simulink model "EPA_Walker"  (R2018a)
settings: Solver=FixedStepDiscrete  StartTime=0.0  StopTime=inf  FixedStep=0.001  RelTol=1e-3  EnableMultiTasking=on
model workspace (MAT data in the model file):
  MCOS : class17 (value not decoded)
undefined symbols (not defined in the file or in its folder): bits_current, bits_GRF, bits_Kd, bits_Kp, bits_position, bits_velocity, deadzone_in_TIB, deadzone_out_TIB, GRF_MAX, GRF_MIN, k_p_TIB, KD_MAX, KD_MIN, KP_MAX, KP_MIN, P_MAX, P_MIN, PressureFilter_CutOffFreq, PressureFilter_Gain, ReadingVoltage, T_MAX, T_MIN, V_MAX, V_MIN, voltageBias_GAS, voltageBias_GL, voltageBias_HAM, voltageBias_IL, voltageBias_POP, voltageBias_RF, voltageBias_SOL, voltageBias_TIB, voltageBias_VAS, voltageMultiplier_GAS, voltageMultiplier_GL, voltageMultiplier_HAM, voltageMultiplier_IL, voltageMultiplier_POP, voltageMultiplier_RF, voltageMultiplier_SOL, voltageMultiplier_TIB, voltageMultiplier_VAS, VoltageResolution
libraries: xpcethercatlib x139, simulink x19, peGeneralControl x18, slrtlib x9
(part 3 of 5)

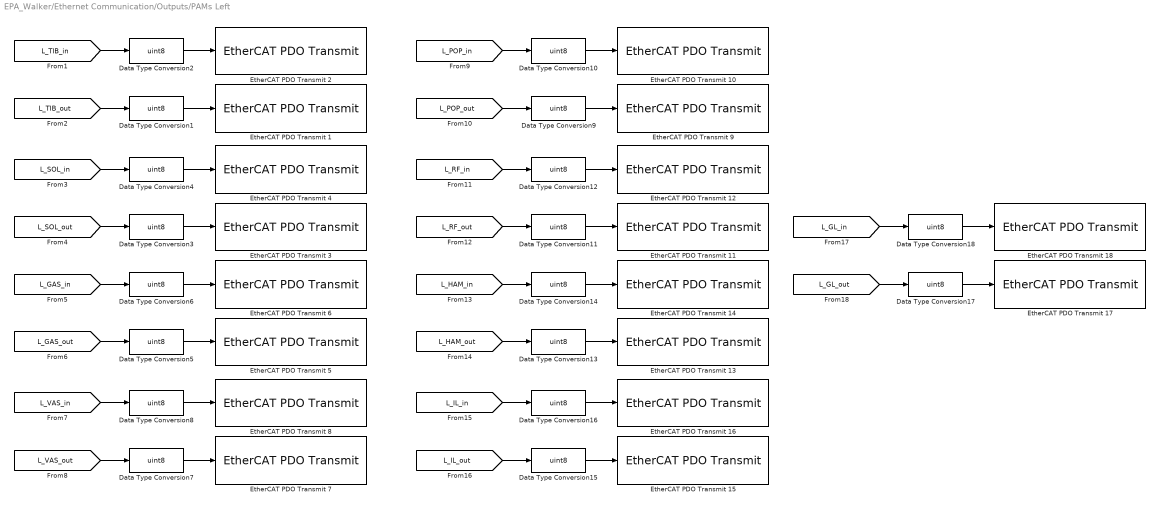
== system EPA_Walker/Ethernet Communication/Outputs/PAMs Left ==
  Data Type Conversion{1..18} (18 alike) : DataTypeConversion  OutDataTypeStr=uint8  RndMeth=Ceiling
  EtherCAT PDO Transmit 1 : xpcethercatlib/EtherCAT PDO Transmit   Priority=3  sig_name=PAMs_L.Outputs.Byte1  sig_offset=1032  sig_type=uint8  type_size=8  sig_dim=1  device_id=0  sample_time=0.001000
      settings: SourceProductName=Simulink Real-Time  SourceProductBaseCode=XP
  EtherCAT PDO Transmit 10 : xpcethercatlib/EtherCAT PDO Transmit   Priority=3  sig_name=PAMs_L.Outputs.Byte8  sig_offset=1088  sig_type=uint8  type_size=8  sig_dim=1  device_id=0  sample_time=0.001000
      settings: SourceProductName=Simulink Real-Time  SourceProductBaseCode=XP
  EtherCAT PDO Transmit 11 : xpcethercatlib/EtherCAT PDO Transmit   Priority=3  sig_name=PAMs_L.Outputs.Byte11  sig_offset=1112  sig_type=uint8  type_size=8  sig_dim=1  device_id=0  sample_time=0.001000
      settings: SourceProductName=Simulink Real-Time  SourceProductBaseCode=XP
  EtherCAT PDO Transmit 12 : xpcethercatlib/EtherCAT PDO Transmit   Priority=3  sig_name=PAMs_L.Outputs.Byte10  sig_offset=1104  sig_type=uint8  type_size=8  sig_dim=1  device_id=0  sample_time=0.001000
      settings: SourceProductName=Simulink Real-Time  SourceProductBaseCode=XP
  EtherCAT PDO Transmit 13 : xpcethercatlib/EtherCAT PDO Transmit   Priority=3  sig_name=PAMs_L.Outputs.Byte13  sig_offset=1128  sig_type=uint8  type_size=8  sig_dim=1  device_id=0  sample_time=0.001000
      settings: SourceProductName=Simulink Real-Time  SourceProductBaseCode=XP
  EtherCAT PDO Transmit 14 : xpcethercatlib/EtherCAT PDO Transmit   Priority=3  sig_name=PAMs_L.Outputs.Byte12  sig_offset=1120  sig_type=uint8  type_size=8  sig_dim=1  device_id=0  sample_time=0.001000
      settings: SourceProductName=Simulink Real-Time  SourceProductBaseCode=XP
  EtherCAT PDO Transmit 15 : xpcethercatlib/EtherCAT PDO Transmit   Priority=3  sig_name=PAMs_L.Outputs.Byte15  sig_offset=1144  sig_type=uint8  type_size=8  sig_dim=1  device_id=0  sample_time=0.001000
      settings: SourceProductName=Simulink Real-Time  SourceProductBaseCode=XP
  EtherCAT PDO Transmit 16 : xpcethercatlib/EtherCAT PDO Transmit   Priority=3  sig_name=PAMs_L.Outputs.Byte14  sig_offset=1136  sig_type=uint8  type_size=8  sig_dim=1  device_id=0  sample_time=0.001000
      settings: SourceProductName=Simulink Real-Time  SourceProductBaseCode=XP
  EtherCAT PDO Transmit 17 : xpcethercatlib/EtherCAT PDO Transmit   Priority=3  sig_name=PAMs_L.Outputs.Byte17  sig_offset=1160  sig_type=uint8  type_size=8  sig_dim=1  device_id=0  sample_time=0.001000
      settings: SourceProductName=Simulink Real-Time  SourceProductBaseCode=XP
  EtherCAT PDO Transmit 18 : xpcethercatlib/EtherCAT PDO Transmit   Priority=3  sig_name=PAMs_L.Outputs.Byte16  sig_offset=1152  sig_type=uint8  type_size=8  sig_dim=1  device_id=0  sample_time=0.001000
      settings: SourceProductName=Simulink Real-Time  SourceProductBaseCode=XP
  EtherCAT PDO Transmit 2 : xpcethercatlib/EtherCAT PDO Transmit   Priority=3  sig_name=PAMs_L.Outputs.Byte0  sig_offset=1024  sig_type=uint8  type_size=8  sig_dim=1  device_id=0  sample_time=0.001000
      settings: SourceProductName=Simulink Real-Time  SourceProductBaseCode=XP
  EtherCAT PDO Transmit 3 : xpcethercatlib/EtherCAT PDO Transmit   Priority=3  sig_name=PAMs_L.Outputs.Byte3  sig_offset=1048  sig_type=uint8  type_size=8  sig_dim=1  device_id=0  sample_time=0.001000
      settings: SourceProductName=Simulink Real-Time  SourceProductBaseCode=XP
  EtherCAT PDO Transmit 4 : xpcethercatlib/EtherCAT PDO Transmit   Priority=3  sig_name=PAMs_L.Outputs.Byte2  sig_offset=1040  sig_type=uint8  type_size=8  sig_dim=1  device_id=0  sample_time=0.001000
      settings: SourceProductName=Simulink Real-Time  SourceProductBaseCode=XP
  EtherCAT PDO Transmit 5 : xpcethercatlib/EtherCAT PDO Transmit   Priority=3  sig_name=PAMs_L.Outputs.Byte5  sig_offset=1064  sig_type=uint8  type_size=8  sig_dim=1  device_id=0  sample_time=0.001000
      settings: SourceProductName=Simulink Real-Time  SourceProductBaseCode=XP
  EtherCAT PDO Transmit 6 : xpcethercatlib/EtherCAT PDO Transmit   Priority=3  sig_name=PAMs_L.Outputs.Byte4  sig_offset=1056  sig_type=uint8  type_size=8  sig_dim=1  device_id=0  sample_time=0.001000
      settings: SourceProductName=Simulink Real-Time  SourceProductBaseCode=XP
  EtherCAT PDO Transmit 7 : xpcethercatlib/EtherCAT PDO Transmit   Priority=3  sig_name=PAMs_L.Outputs.Byte7  sig_offset=1080  sig_type=uint8  type_size=8  sig_dim=1  device_id=0  sample_time=0.001000
      settings: SourceProductName=Simulink Real-Time  SourceProductBaseCode=XP
  EtherCAT PDO Transmit 8 : xpcethercatlib/EtherCAT PDO Transmit   Priority=3  sig_name=PAMs_L.Outputs.Byte6  sig_offset=1072  sig_type=uint8  type_size=8  sig_dim=1  device_id=0  sample_time=0.001000
      settings: SourceProductName=Simulink Real-Time  SourceProductBaseCode=XP
  EtherCAT PDO Transmit 9 : xpcethercatlib/EtherCAT PDO Transmit   Priority=3  sig_name=PAMs_L.Outputs.Byte9  sig_offset=1096  sig_type=uint8  type_size=8  sig_dim=1  device_id=0  sample_time=0.001000
      settings: SourceProductName=Simulink Real-Time  SourceProductBaseCode=XP
  wires:
  Data Type Conversion2/1 -> EtherCAT PDO Transmit 2/1
  [L_TIB_in] -> Data Type Conversion2/1
  [L_TIB_out] -> Data Type Conversion1/1
  Data Type Conversion1/1 -> EtherCAT PDO Transmit 1/1
  Data Type Conversion3/1 -> EtherCAT PDO Transmit 3/1
  [L_SOL_in] -> Data Type Conversion4/1
  [L_SOL_out] -> Data Type Conversion3/1
  Data Type Conversion4/1 -> EtherCAT PDO Transmit 4/1
  Data Type Conversion6/1 -> EtherCAT PDO Transmit 6/1
  Data Type Conversion8/1 -> EtherCAT PDO Transmit 8/1
  [L_VAS_out] -> Data Type Conversion7/1
  [L_GAS_in] -> Data Type Conversion6/1
  [L_GAS_out] -> Data Type Conversion5/1
  [L_VAS_in] -> Data Type Conversion8/1
  Data Type Conversion7/1 -> EtherCAT PDO Transmit 7/1
  Data Type Conversion5/1 -> EtherCAT PDO Transmit 5/1
  [L_IL_in] -> Data Type Conversion16/1
  Data Type Conversion16/1 -> EtherCAT PDO Transmit 16/1
  Data Type Conversion13/1 -> EtherCAT PDO Transmit 13/1
  [L_HAM_out] -> Data Type Conversion13/1
  [L_IL_out] -> Data Type Conversion15/1
  [L_HAM_in] -> Data Type Conversion14/1
  Data Type Conversion14/1 -> EtherCAT PDO Transmit 14/1
  Data Type Conversion10/1 -> EtherCAT PDO Transmit 10/1
  Data Type Conversion12/1 -> EtherCAT PDO Transmit 12/1
  [L_RF_out] -> Data Type Conversion11/1
  [L_POP_in] -> Data Type Conversion10/1
  Data Type Conversion15/1 -> EtherCAT PDO Transmit 15/1
  [L_POP_out] -> Data Type Conversion9/1
  [L_RF_in] -> Data Type Conversion12/1
  Data Type Conversion11/1 -> EtherCAT PDO Transmit 11/1
  Data Type Conversion9/1 -> EtherCAT PDO Transmit 9/1
  Data Type Conversion17/1 -> EtherCAT PDO Transmit 17/1
  [L_GL_in] -> Data Type Conversion18/1
  [L_GL_out] -> Data Type Conversion17/1
  Data Type Conversion18/1 -> EtherCAT PDO Transmit 18/1

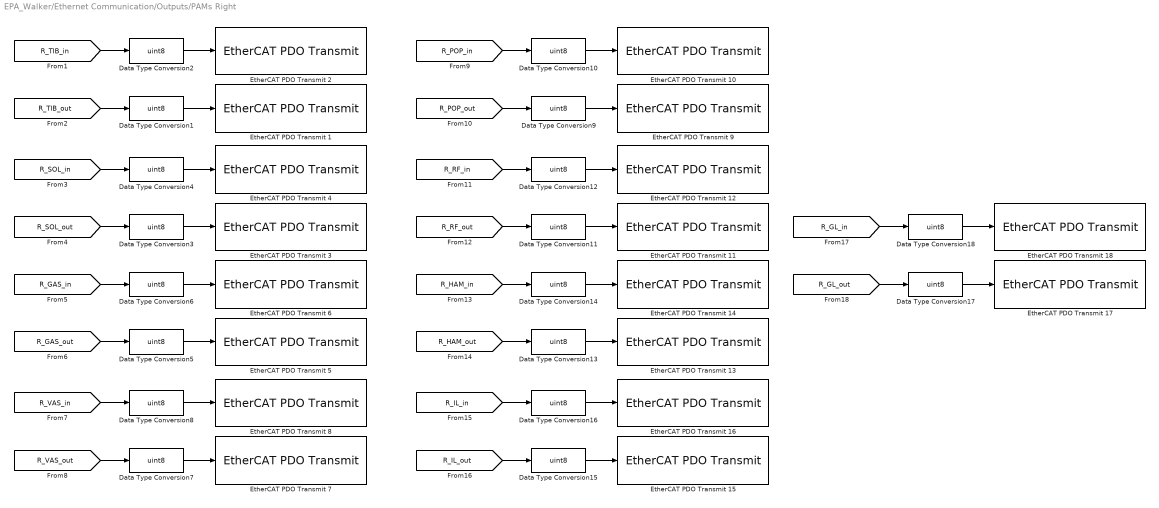
== system EPA_Walker/Ethernet Communication/Outputs/PAMs Right ==
  Data Type Conversion{1..18} (18 alike) : DataTypeConversion  OutDataTypeStr=uint8  RndMeth=Ceiling
  EtherCAT PDO Transmit 1 : xpcethercatlib/EtherCAT PDO Transmit   Priority=3  sig_name=PAMs_R.Outputs.Byte1  sig_offset=520  sig_type=uint8  type_size=8  sig_dim=1  device_id=0  sample_time=0.001000
      settings: SourceProductName=Simulink Real-Time  SourceProductBaseCode=XP
  EtherCAT PDO Transmit 10 : xpcethercatlib/EtherCAT PDO Transmit   Priority=3  sig_name=PAMs_R.Outputs.Byte8  sig_offset=576  sig_type=uint8  type_size=8  sig_dim=1  device_id=0  sample_time=0.001000
      settings: SourceProductName=Simulink Real-Time  SourceProductBaseCode=XP
  EtherCAT PDO Transmit 11 : xpcethercatlib/EtherCAT PDO Transmit   Priority=3  sig_name=PAMs_R.Outputs.Byte11  sig_offset=600  sig_type=uint8  type_size=8  sig_dim=1  device_id=0  sample_time=0.001000
      settings: SourceProductName=Simulink Real-Time  SourceProductBaseCode=XP
  EtherCAT PDO Transmit 12 : xpcethercatlib/EtherCAT PDO Transmit   Priority=3  sig_name=PAMs_R.Outputs.Byte10  sig_offset=592  sig_type=uint8  type_size=8  sig_dim=1  device_id=0  sample_time=0.001000
      settings: SourceProductName=Simulink Real-Time  SourceProductBaseCode=XP
  EtherCAT PDO Transmit 13 : xpcethercatlib/EtherCAT PDO Transmit   Priority=3  sig_name=PAMs_R.Outputs.Byte13  sig_offset=616  sig_type=uint8  type_size=8  sig_dim=1  device_id=0  sample_time=0.001000
      settings: SourceProductName=Simulink Real-Time  SourceProductBaseCode=XP
  EtherCAT PDO Transmit 14 : xpcethercatlib/EtherCAT PDO Transmit   Priority=3  sig_name=PAMs_R.Outputs.Byte12  sig_offset=608  sig_type=uint8  type_size=8  sig_dim=1  device_id=0  sample_time=0.001000
      settings: SourceProductName=Simulink Real-Time  SourceProductBaseCode=XP
  EtherCAT PDO Transmit 15 : xpcethercatlib/EtherCAT PDO Transmit   Priority=3  sig_name=PAMs_R.Outputs.Byte15  sig_offset=632  sig_type=uint8  type_size=8  sig_dim=1  device_id=0  sample_time=0.001000
      settings: SourceProductName=Simulink Real-Time  SourceProductBaseCode=XP
  EtherCAT PDO Transmit 16 : xpcethercatlib/EtherCAT PDO Transmit   Priority=3  sig_name=PAMs_R.Outputs.Byte14  sig_offset=624  sig_type=uint8  type_size=8  sig_dim=1  device_id=0  sample_time=0.001000
      settings: SourceProductName=Simulink Real-Time  SourceProductBaseCode=XP
  EtherCAT PDO Transmit 17 : xpcethercatlib/EtherCAT PDO Transmit   Priority=3  sig_name=PAMs_R.Outputs.Byte17  sig_offset=648  sig_type=uint8  type_size=8  sig_dim=1  device_id=0  sample_time=0.001000
      settings: SourceProductName=Simulink Real-Time  SourceProductBaseCode=XP
  EtherCAT PDO Transmit 18 : xpcethercatlib/EtherCAT PDO Transmit   Priority=3  sig_name=PAMs_R.Outputs.Byte16  sig_offset=640  sig_type=uint8  type_size=8  sig_dim=1  device_id=0  sample_time=0.001000
      settings: SourceProductName=Simulink Real-Time  SourceProductBaseCode=XP
  EtherCAT PDO Transmit 2 : xpcethercatlib/EtherCAT PDO Transmit   Priority=3  sig_name=PAMs_R.Outputs.Byte0  sig_offset=512  sig_type=uint8  type_size=8  sig_dim=1  device_id=0  sample_time=0.001000
      settings: SourceProductName=Simulink Real-Time  SourceProductBaseCode=XP
  EtherCAT PDO Transmit 3 : xpcethercatlib/EtherCAT PDO Transmit   Priority=3  sig_name=PAMs_R.Outputs.Byte3  sig_offset=536  sig_type=uint8  type_size=8  sig_dim=1  device_id=0  sample_time=0.001000
      settings: SourceProductName=Simulink Real-Time  SourceProductBaseCode=XP
  EtherCAT PDO Transmit 4 : xpcethercatlib/EtherCAT PDO Transmit   Priority=3  sig_name=PAMs_R.Outputs.Byte2  sig_offset=528  sig_type=uint8  type_size=8  sig_dim=1  device_id=0  sample_time=0.001000
      settings: SourceProductName=Simulink Real-Time  SourceProductBaseCode=XP
  EtherCAT PDO Transmit 5 : xpcethercatlib/EtherCAT PDO Transmit   Priority=3  sig_name=PAMs_R.Outputs.Byte5  sig_offset=552  sig_type=uint8  type_size=8  sig_dim=1  device_id=0  sample_time=0.001000
      settings: SourceProductName=Simulink Real-Time  SourceProductBaseCode=XP
  EtherCAT PDO Transmit 6 : xpcethercatlib/EtherCAT PDO Transmit   Priority=3  sig_name=PAMs_R.Outputs.Byte4  sig_offset=544  sig_type=uint8  type_size=8  sig_dim=1  device_id=0  sample_time=0.001000
      settings: SourceProductName=Simulink Real-Time  SourceProductBaseCode=XP
  EtherCAT PDO Transmit 7 : xpcethercatlib/EtherCAT PDO Transmit   Priority=3  sig_name=PAMs_R.Outputs.Byte7  sig_offset=568  sig_type=uint8  type_size=8  sig_dim=1  device_id=0  sample_time=0.001000
      settings: SourceProductName=Simulink Real-Time  SourceProductBaseCode=XP
  EtherCAT PDO Transmit 8 : xpcethercatlib/EtherCAT PDO Transmit   Priority=3  sig_name=PAMs_R.Outputs.Byte6  sig_offset=560  sig_type=uint8  type_size=8  sig_dim=1  device_id=0  sample_time=0.001000
      settings: SourceProductName=Simulink Real-Time  SourceProductBaseCode=XP
  EtherCAT PDO Transmit 9 : xpcethercatlib/EtherCAT PDO Transmit   Priority=3  sig_name=PAMs_R.Outputs.Byte9  sig_offset=584  sig_type=uint8  type_size=8  sig_dim=1  device_id=0  sample_time=0.001000
      settings: SourceProductName=Simulink Real-Time  SourceProductBaseCode=XP
  wires:
  Data Type Conversion2/1 -> EtherCAT PDO Transmit 2/1
  [R_TIB_in] -> Data Type Conversion2/1
  [R_TIB_out] -> Data Type Conversion1/1
  Data Type Conversion1/1 -> EtherCAT PDO Transmit 1/1
  Data Type Conversion3/1 -> EtherCAT PDO Transmit 3/1
  [R_SOL_in] -> Data Type Conversion4/1
  [R_SOL_out] -> Data Type Conversion3/1
  Data Type Conversion4/1 -> EtherCAT PDO Transmit 4/1
  Data Type Conversion6/1 -> EtherCAT PDO Transmit 6/1
  Data Type Conversion8/1 -> EtherCAT PDO Transmit 8/1
  [R_VAS_out] -> Data Type Conversion7/1
  [R_GAS_in] -> Data Type Conversion6/1
  [R_GAS_out] -> Data Type Conversion5/1
  [R_VAS_in] -> Data Type Conversion8/1
  Data Type Conversion7/1 -> EtherCAT PDO Transmit 7/1
  Data Type Conversion5/1 -> EtherCAT PDO Transmit 5/1
  [R_IL_in] -> Data Type Conversion16/1
  Data Type Conversion16/1 -> EtherCAT PDO Transmit 16/1
  Data Type Conversion13/1 -> EtherCAT PDO Transmit 13/1
  [R_HAM_out] -> Data Type Conversion13/1
  [R_IL_out] -> Data Type Conversion15/1
  [R_HAM_in] -> Data Type Conversion14/1
  Data Type Conversion14/1 -> EtherCAT PDO Transmit 14/1
  Data Type Conversion10/1 -> EtherCAT PDO Transmit 10/1
  Data Type Conversion12/1 -> EtherCAT PDO Transmit 12/1
  [R_RF_out] -> Data Type Conversion11/1
  [R_POP_in] -> Data Type Conversion10/1
  Data Type Conversion15/1 -> EtherCAT PDO Transmit 15/1
  [R_POP_out] -> Data Type Conversion9/1
  [R_RF_in] -> Data Type Conversion12/1
  Data Type Conversion11/1 -> EtherCAT PDO Transmit 11/1
  Data Type Conversion9/1 -> EtherCAT PDO Transmit 9/1
  Data Type Conversion17/1 -> EtherCAT PDO Transmit 17/1
  [R_GL_in] -> Data Type Conversion18/1
  [R_GL_out] -> Data Type Conversion17/1
  Data Type Conversion18/1 -> EtherCAT PDO Transmit 18/1

== system EPA_Walker/High Level Control/HL Left/Stance phase ==
  "GRFz " : Inport
  Knee : Inport  Port=2
  C_Knee : Inport  Port=3
  Phi_0_Knee : Inport  Port=4
  Hip_Torque_Stance : Inport  Port=5
  Hip : Inport  Port=6
  C_Hip : Inport  Port=7
  Phi_0_Hip : Inport  Port=8
  FMCH Enable : Inport  Port=9
  Enable : EnablePort  StatesWhenEnabling=reset
  FMCH (Static) : Subsystem
  FMCK (Static) : Subsystem
  Switch : Switch  Threshold=1
  Hip_torque_HL : Outport
  Knee_torque_HL : Outport  Port=2
  wires:
  "GRFz "/1 -> FMCK (Static)/1(GRF_Z), FMCH (Static)/1(GRF_Z)
  Knee/1 -> FMCK (Static)/2(angKne)
  FMCK (Static)/1(torMotKne) -> Knee_torque_HL/1
  Hip_Torque_Stance/1 -> Switch/3
  C_Knee/1 -> FMCK (Static)/3(C_)
  Phi_0_Knee/1 -> FMCK (Static)/4(Phi_0)
  C_Hip/1 -> FMCH (Static)/3(C_Hip)
  Phi_0_Hip/1 -> FMCH (Static)/4(Phi_0_Hip)
  FMCH (Static)/1(torMotHip) -> Switch/1
  Hip/1 -> FMCH (Static)/2(angHip)
  Switch/1 -> Hip_torque_HL/1
  FMCH Enable/1 -> Switch/2

== system EPA_Walker/High Level Control/HL Left/Swing phase ==
  Hip_Position_Des_swing : Inport
  Knee_Position_Des_swing : Inport  Port=2
  Enable : EnablePort  StatesWhenEnabling=reset
  Hip : Outport
  Knee : Outport  Port=2
  wires:
  Hip_Position_Des_swing/1 -> Hip/1
  Knee_Position_Des_swing/1 -> Knee/1

== system EPA_Walker/High Level Control/HL Right/Stance phase ==
  "GRFz " : Inport
  Knee : Inport  Port=2
  C_Knee : Inport  Port=3
  Phi_0_Knee : Inport  Port=4
  Hip_Torque_Stance : Inport  Port=5
  Hip : Inport  Port=6
  C_Hip : Inport  Port=7
  Phi_0_Hip : Inport  Port=8
  FMCH Enable : Inport  Port=9
  Enable : EnablePort  StatesWhenEnabling=reset
  FMCH (Static) : Subsystem
  FMCK (Static) : Subsystem
  Switch : Switch  Threshold=1
  Hip_torque_HL : Outport
  Knee_torque_HL : Outport  Port=2
  wires:
  "GRFz "/1 -> FMCK (Static)/1(GRF_Z), FMCH (Static)/1(GRF_Z)
  Knee/1 -> FMCK (Static)/2(angKne)
  FMCK (Static)/1(torMotKne) -> Knee_torque_HL/1
  Hip_Torque_Stance/1 -> Switch/3
  C_Knee/1 -> FMCK (Static)/3(C_)
  Phi_0_Knee/1 -> FMCK (Static)/4(Phi_0)
  C_Hip/1 -> FMCH (Static)/3(C_Hip)
  Phi_0_Hip/1 -> FMCH (Static)/4(Phi_0_Hip)
  FMCH (Static)/1(torMotHip) -> Switch/1
  Hip/1 -> FMCH (Static)/2(angHip)
  Switch/1 -> Hip_torque_HL/1
  FMCH Enable/1 -> Switch/2

== system EPA_Walker/High Level Control/HL Right/Swing phase ==
  Hip_Position_Des_flight : Inport
  Knee_Position_Des_flight : Inport  Port=2
  Enable : EnablePort  StatesWhenEnabling=reset
  Hip : Outport
  Knee : Outport  Port=2
  wires:
  Hip_Position_Des_flight/1 -> Hip/1
  Knee_Position_Des_flight/1 -> Knee/1

== system EPA_Walker/PAMs/PAMs Left/GAS ==
  Pressure Des : Inport
  Delay : Delay  DelayLength=1
  PID Controller : simulink/Continuous/PID Controller  Controller=PID  TimeDomain=Discrete-time  SampleTime=-1  IntegratorMethod=Forward Euler  FilterMethod=Forward Euler  Form=Ideal  UseFilter=on  ControllerParametersSource=external  P=k_p_pam  I=0  D=0.45*0.15/8  N=100  InitialConditionSource=internal  InitialConditionForIntegrator=0  InitialConditionForFilter=0  ExternalReset=none  LimitOutput=off  UpperSaturationLimit=inf  LowerSaturationLimit=-inf  LinearizeAsGain=on  AntiWindupMode=none  Kb=1  TrackingMode=off  Kt=1  PParamMin=[]  PParamMax=[]  IParamMin=[]  IParamMax=[]  DParamMin=[]  DParamMax=[]  NParamMin=[]  NParamMax=[]  KbParamMin=[]  KbParamMax=[]  KtParamMin=[]  KtParamMax=[]  POutMin=[]  POutMax=[]  IOutMin=[]  IOutMax=[]  DOutMin=[]  DOutMax=[]  NOutMin=[]  NOutMax=[]  KbOutMin=[]  KbOutMax=[]  KtOutMin=[]  KtOutMax=[]  IntegratorOutMin=[]  IntegratorOutMax=[]  FilterOutMin=[]  FilterOutMax=[]  SumOutMin=[]  SumOutMax=[]  SumI1OutMin=[]  SumI1OutMax=[]  SumI2OutMin=[]  SumI2OutMax=[]  SumI3OutMin=[]  SumI3OutMax=[]  SumDOutMin=[]  SumDOutMax=[]  SaturationOutMin=[]  SaturationOutMax=[]  IntegratorContinuousStateAttributes=''  IntegratorStateMustResolveToSignalObject=off  IntegratorRTWStateStorageClass=Auto  FilterContinuousStateAttributes=''  FilterStateMustResolveToSignalObject=off  FilterRTWStateStorageClass=Auto  DifferentiatorICPrevScaledInput=0  DifferentiatorOutMin=[]  DifferentiatorOutMax=[]  FilterDiffOutCoefMin=[]  FilterDiffOutCoefMax=[]  SumDenOutMin=[]  SumDenOutMax=[]  SumNumOutMin=[]  SumNumOutMax=[]  ReciprocalOutMin=[]  ReciprocalOutMax=[]  DivideOutMin=[]  DivideOutMax=[]  TunerSelectOption=Transfer Function Based (PID Tuner App)
  Solenoids : MATLAB Function  TreatAsAtomicUnit=on
  Sum : Sum  Inputs=|+-
  tag scope: L_GAS_in=global, L_GAS_out=global
  wires:
  Solenoids/3(inside_deadzone_1) -> Delay/1
  Delay/1 -> Solenoids/2(inside_deadzone)
  Pressure Des/1 -> Sum/1
  [L_GAS_pres] -> Sum/2
  [L_deadzone_in] -> Solenoids/3(deadzone_in)
  [L_deadzone_out] -> Solenoids/4(deadzone_out)
  Solenoids/1(intake) -> [L_GAS_in]
  Solenoids/2(outtake) -> [L_GAS_out]
  [L_k_i] -> PID Controller/3
  [L_k_d] -> PID Controller/4
  [L_N] -> PID Controller/5
  Sum/1 -> PID Controller/1
  PID Controller/1 -> Solenoids/1(control)
  [L_k_p] -> PID Controller/2
  [L_PAMs_off] -> Solenoids/5(PAMs_on)
  [System_on] -> Solenoids/6(System_on)
  [L_Depressurize_PAMs] -> Solenoids/7(depressurize)

== system EPA_Walker/PAMs/PAMs Left/GL ==
  Pressure Des : Inport
  Delay : Delay  DelayLength=1
  PID Controller : simulink/Continuous/PID Controller  Controller=PID  TimeDomain=Discrete-time  SampleTime=-1  IntegratorMethod=Forward Euler  FilterMethod=Forward Euler  Form=Ideal  UseFilter=on  ControllerParametersSource=external  P=k_p_pam  I=0  D=0.45*0.15/8  N=100  InitialConditionSource=internal  InitialConditionForIntegrator=0  InitialConditionForFilter=0  ExternalReset=none  LimitOutput=off  UpperSaturationLimit=inf  LowerSaturationLimit=-inf  LinearizeAsGain=on  AntiWindupMode=none  Kb=1  TrackingMode=off  Kt=1  PParamMin=[]  PParamMax=[]  IParamMin=[]  IParamMax=[]  DParamMin=[]  DParamMax=[]  NParamMin=[]  NParamMax=[]  KbParamMin=[]  KbParamMax=[]  KtParamMin=[]  KtParamMax=[]  POutMin=[]  POutMax=[]  IOutMin=[]  IOutMax=[]  DOutMin=[]  DOutMax=[]  NOutMin=[]  NOutMax=[]  KbOutMin=[]  KbOutMax=[]  KtOutMin=[]  KtOutMax=[]  IntegratorOutMin=[]  IntegratorOutMax=[]  FilterOutMin=[]  FilterOutMax=[]  SumOutMin=[]  SumOutMax=[]  SumI1OutMin=[]  SumI1OutMax=[]  SumI2OutMin=[]  SumI2OutMax=[]  SumI3OutMin=[]  SumI3OutMax=[]  SumDOutMin=[]  SumDOutMax=[]  SaturationOutMin=[]  SaturationOutMax=[]  IntegratorContinuousStateAttributes=''  IntegratorStateMustResolveToSignalObject=off  IntegratorRTWStateStorageClass=Auto  FilterContinuousStateAttributes=''  FilterStateMustResolveToSignalObject=off  FilterRTWStateStorageClass=Auto  DifferentiatorICPrevScaledInput=0  DifferentiatorOutMin=[]  DifferentiatorOutMax=[]  FilterDiffOutCoefMin=[]  FilterDiffOutCoefMax=[]  SumDenOutMin=[]  SumDenOutMax=[]  SumNumOutMin=[]  SumNumOutMax=[]  ReciprocalOutMin=[]  ReciprocalOutMax=[]  DivideOutMin=[]  DivideOutMax=[]  TunerSelectOption=Transfer Function Based (PID Tuner App)
  Solenoids : MATLAB Function  TreatAsAtomicUnit=on
  Sum : Sum  Inputs=|+-
  tag scope: L_GL_in=global, L_GL_out=global
  wires:
  Solenoids/3(inside_deadzone_1) -> Delay/1
  Delay/1 -> Solenoids/2(inside_deadzone)
  Pressure Des/1 -> Sum/1
  [L_GL_pres] -> Sum/2
  [L_deadzone_in] -> Solenoids/3(deadzone_in)
  [L_deadzone_out] -> Solenoids/4(deadzone_out)
  Solenoids/1(intake) -> [L_GL_in]
  Solenoids/2(outtake) -> [L_GL_out]
  [L_k_i] -> PID Controller/3
  [L_k_d] -> PID Controller/4
  [L_N] -> PID Controller/5
  Sum/1 -> PID Controller/1
  PID Controller/1 -> Solenoids/1(control)
  [L_k_p] -> PID Controller/2
  [L_PAMs_off] -> Solenoids/5(PAMs_on)
  [System_on] -> Solenoids/6(System_on)
  [L_Depressurize_PAMs] -> Solenoids/7(depressurize)

== system EPA_Walker/PAMs/PAMs Left/HAM ==
  Pressure Des : Inport
  Delay : Delay  DelayLength=1
  PID Controller : simulink/Continuous/PID Controller  Controller=PID  TimeDomain=Discrete-time  SampleTime=-1  IntegratorMethod=Forward Euler  FilterMethod=Forward Euler  Form=Ideal  UseFilter=on  ControllerParametersSource=external  P=k_p_pam  I=0  D=0.45*0.15/8  N=100  InitialConditionSource=internal  InitialConditionForIntegrator=0  InitialConditionForFilter=0  ExternalReset=none  LimitOutput=off  UpperSaturationLimit=inf  LowerSaturationLimit=-inf  LinearizeAsGain=on  AntiWindupMode=none  Kb=1  TrackingMode=off  Kt=1  PParamMin=[]  PParamMax=[]  IParamMin=[]  IParamMax=[]  DParamMin=[]  DParamMax=[]  NParamMin=[]  NParamMax=[]  KbParamMin=[]  KbParamMax=[]  KtParamMin=[]  KtParamMax=[]  POutMin=[]  POutMax=[]  IOutMin=[]  IOutMax=[]  DOutMin=[]  DOutMax=[]  NOutMin=[]  NOutMax=[]  KbOutMin=[]  KbOutMax=[]  KtOutMin=[]  KtOutMax=[]  IntegratorOutMin=[]  IntegratorOutMax=[]  FilterOutMin=[]  FilterOutMax=[]  SumOutMin=[]  SumOutMax=[]  SumI1OutMin=[]  SumI1OutMax=[]  SumI2OutMin=[]  SumI2OutMax=[]  SumI3OutMin=[]  SumI3OutMax=[]  SumDOutMin=[]  SumDOutMax=[]  SaturationOutMin=[]  SaturationOutMax=[]  IntegratorContinuousStateAttributes=''  IntegratorStateMustResolveToSignalObject=off  IntegratorRTWStateStorageClass=Auto  FilterContinuousStateAttributes=''  FilterStateMustResolveToSignalObject=off  FilterRTWStateStorageClass=Auto  DifferentiatorICPrevScaledInput=0  DifferentiatorOutMin=[]  DifferentiatorOutMax=[]  FilterDiffOutCoefMin=[]  FilterDiffOutCoefMax=[]  SumDenOutMin=[]  SumDenOutMax=[]  SumNumOutMin=[]  SumNumOutMax=[]  ReciprocalOutMin=[]  ReciprocalOutMax=[]  DivideOutMin=[]  DivideOutMax=[]  TunerSelectOption=Transfer Function Based (PID Tuner App)
  Solenoids : MATLAB Function  TreatAsAtomicUnit=on
  Sum : Sum  Inputs=|+-
  tag scope: L_HAM_in=global, L_HAM_out=global
  wires:
  Solenoids/3(inside_deadzone_1) -> Delay/1
  Delay/1 -> Solenoids/2(inside_deadzone)
  Pressure Des/1 -> Sum/1
  [L_HAM_pres] -> Sum/2
  [L_deadzone_in] -> Solenoids/3(deadzone_in)
  [L_deadzone_out] -> Solenoids/4(deadzone_out)
  Solenoids/1(intake) -> [L_HAM_in]
  Solenoids/2(outtake) -> [L_HAM_out]
  [L_k_i] -> PID Controller/3
  [L_k_d] -> PID Controller/4
  [L_N] -> PID Controller/5
  Sum/1 -> PID Controller/1
  PID Controller/1 -> Solenoids/1(control)
  [L_k_p] -> PID Controller/2
  [L_PAMs_off] -> Solenoids/5(PAMs_on)
  [System_on] -> Solenoids/6(System_on)
  [L_Depressurize_PAMs] -> Solenoids/7(depressurize)

== system EPA_Walker/PAMs/PAMs Left/IL ==
  Pressure Des : Inport
  Delay : Delay  DelayLength=1
  PID Controller : simulink/Continuous/PID Controller  Controller=PID  TimeDomain=Discrete-time  SampleTime=-1  IntegratorMethod=Forward Euler  FilterMethod=Forward Euler  Form=Ideal  UseFilter=on  ControllerParametersSource=external  P=k_p_pam  I=0  D=0.45*0.15/8  N=100  InitialConditionSource=internal  InitialConditionForIntegrator=0  InitialConditionForFilter=0  ExternalReset=none  LimitOutput=off  UpperSaturationLimit=inf  LowerSaturationLimit=-inf  LinearizeAsGain=on  AntiWindupMode=none  Kb=1  TrackingMode=off  Kt=1  PParamMin=[]  PParamMax=[]  IParamMin=[]  IParamMax=[]  DParamMin=[]  DParamMax=[]  NParamMin=[]  NParamMax=[]  KbParamMin=[]  KbParamMax=[]  KtParamMin=[]  KtParamMax=[]  POutMin=[]  POutMax=[]  IOutMin=[]  IOutMax=[]  DOutMin=[]  DOutMax=[]  NOutMin=[]  NOutMax=[]  KbOutMin=[]  KbOutMax=[]  KtOutMin=[]  KtOutMax=[]  IntegratorOutMin=[]  IntegratorOutMax=[]  FilterOutMin=[]  FilterOutMax=[]  SumOutMin=[]  SumOutMax=[]  SumI1OutMin=[]  SumI1OutMax=[]  SumI2OutMin=[]  SumI2OutMax=[]  SumI3OutMin=[]  SumI3OutMax=[]  SumDOutMin=[]  SumDOutMax=[]  SaturationOutMin=[]  SaturationOutMax=[]  IntegratorContinuousStateAttributes=''  IntegratorStateMustResolveToSignalObject=off  IntegratorRTWStateStorageClass=Auto  FilterContinuousStateAttributes=''  FilterStateMustResolveToSignalObject=off  FilterRTWStateStorageClass=Auto  DifferentiatorICPrevScaledInput=0  DifferentiatorOutMin=[]  DifferentiatorOutMax=[]  FilterDiffOutCoefMin=[]  FilterDiffOutCoefMax=[]  SumDenOutMin=[]  SumDenOutMax=[]  SumNumOutMin=[]  SumNumOutMax=[]  ReciprocalOutMin=[]  ReciprocalOutMax=[]  DivideOutMin=[]  DivideOutMax=[]  TunerSelectOption=Transfer Function Based (PID Tuner App)
  Solenoids : MATLAB Function  TreatAsAtomicUnit=on
  Sum : Sum  Inputs=|+-
  tag scope: L_IL_in=global, L_IL_out=global
  wires:
  Solenoids/3(inside_deadzone_1) -> Delay/1
  Delay/1 -> Solenoids/2(inside_deadzone)
  Pressure Des/1 -> Sum/1
  [L_IL_pres] -> Sum/2
  [L_deadzone_in] -> Solenoids/3(deadzone_in)
  [L_deadzone_out] -> Solenoids/4(deadzone_out)
  Solenoids/1(intake) -> [L_IL_in]
  Solenoids/2(outtake) -> [L_IL_out]
  [L_k_i] -> PID Controller/3
  [L_k_d] -> PID Controller/4
  [L_N] -> PID Controller/5
  Sum/1 -> PID Controller/1
  PID Controller/1 -> Solenoids/1(control)
  [L_k_p] -> PID Controller/2
  [L_PAMs_off] -> Solenoids/5(PAMs_on)
  [System_on] -> Solenoids/6(System_on)
  [L_Depressurize_PAMs] -> Solenoids/7(depressurize)

== system EPA_Walker/PAMs/PAMs Left/POP ==
  Pressure Des : Inport
  Delay : Delay  DelayLength=1
  PID Controller : simulink/Continuous/PID Controller  Controller=PID  TimeDomain=Discrete-time  SampleTime=-1  IntegratorMethod=Forward Euler  FilterMethod=Forward Euler  Form=Ideal  UseFilter=on  ControllerParametersSource=external  P=k_p_pam  I=0  D=0.45*0.15/8  N=100  InitialConditionSource=internal  InitialConditionForIntegrator=0  InitialConditionForFilter=0  ExternalReset=none  LimitOutput=off  UpperSaturationLimit=inf  LowerSaturationLimit=-inf  LinearizeAsGain=on  AntiWindupMode=none  Kb=1  TrackingMode=off  Kt=1  PParamMin=[]  PParamMax=[]  IParamMin=[]  IParamMax=[]  DParamMin=[]  DParamMax=[]  NParamMin=[]  NParamMax=[]  KbParamMin=[]  KbParamMax=[]  KtParamMin=[]  KtParamMax=[]  POutMin=[]  POutMax=[]  IOutMin=[]  IOutMax=[]  DOutMin=[]  DOutMax=[]  NOutMin=[]  NOutMax=[]  KbOutMin=[]  KbOutMax=[]  KtOutMin=[]  KtOutMax=[]  IntegratorOutMin=[]  IntegratorOutMax=[]  FilterOutMin=[]  FilterOutMax=[]  SumOutMin=[]  SumOutMax=[]  SumI1OutMin=[]  SumI1OutMax=[]  SumI2OutMin=[]  SumI2OutMax=[]  SumI3OutMin=[]  SumI3OutMax=[]  SumDOutMin=[]  SumDOutMax=[]  SaturationOutMin=[]  SaturationOutMax=[]  IntegratorContinuousStateAttributes=''  IntegratorStateMustResolveToSignalObject=off  IntegratorRTWStateStorageClass=Auto  FilterContinuousStateAttributes=''  FilterStateMustResolveToSignalObject=off  FilterRTWStateStorageClass=Auto  DifferentiatorICPrevScaledInput=0  DifferentiatorOutMin=[]  DifferentiatorOutMax=[]  FilterDiffOutCoefMin=[]  FilterDiffOutCoefMax=[]  SumDenOutMin=[]  SumDenOutMax=[]  SumNumOutMin=[]  SumNumOutMax=[]  ReciprocalOutMin=[]  ReciprocalOutMax=[]  DivideOutMin=[]  DivideOutMax=[]  TunerSelectOption=Transfer Function Based (PID Tuner App)
  Solenoids : MATLAB Function  TreatAsAtomicUnit=on
  Sum : Sum  Inputs=|+-
  tag scope: L_POP_in=global, L_POP_out=global
  wires:
  Solenoids/3(inside_deadzone_1) -> Delay/1
  Delay/1 -> Solenoids/2(inside_deadzone)
  Pressure Des/1 -> Sum/1
  [L_POP_pres] -> Sum/2
  [L_deadzone_in_pop] -> Solenoids/3(deadzone_in)
  [L_deadzone_out_pop] -> Solenoids/4(deadzone_out)
  Solenoids/1(intake) -> [L_POP_in]
  Solenoids/2(outtake) -> [L_POP_out]
  [L_k_i] -> PID Controller/3
  [L_k_d] -> PID Controller/4
  [L_N] -> PID Controller/5
  Sum/1 -> PID Controller/1
  PID Controller/1 -> Solenoids/1(control)
  [L_k_p] -> PID Controller/2
  [L_PAMs_off] -> Solenoids/5(PAMs_on)
  [System_on] -> Solenoids/6(System_on)
  [L_Depressurize_PAMs] -> Solenoids/7(depressurize)

== system EPA_Walker/PAMs/PAMs Left/RF ==
  Pressure Des : Inport
  Delay : Delay  DelayLength=1
  PID Controller : simulink/Continuous/PID Controller  Controller=PID  TimeDomain=Discrete-time  SampleTime=-1  IntegratorMethod=Forward Euler  FilterMethod=Forward Euler  Form=Ideal  UseFilter=on  ControllerParametersSource=external  P=k_p_pam  I=0  D=0.45*0.15/8  N=100  InitialConditionSource=internal  InitialConditionForIntegrator=0  InitialConditionForFilter=0  ExternalReset=none  LimitOutput=off  UpperSaturationLimit=inf  LowerSaturationLimit=-inf  LinearizeAsGain=on  AntiWindupMode=none  Kb=1  TrackingMode=off  Kt=1  PParamMin=[]  PParamMax=[]  IParamMin=[]  IParamMax=[]  DParamMin=[]  DParamMax=[]  NParamMin=[]  NParamMax=[]  KbParamMin=[]  KbParamMax=[]  KtParamMin=[]  KtParamMax=[]  POutMin=[]  POutMax=[]  IOutMin=[]  IOutMax=[]  DOutMin=[]  DOutMax=[]  NOutMin=[]  NOutMax=[]  KbOutMin=[]  KbOutMax=[]  KtOutMin=[]  KtOutMax=[]  IntegratorOutMin=[]  IntegratorOutMax=[]  FilterOutMin=[]  FilterOutMax=[]  SumOutMin=[]  SumOutMax=[]  SumI1OutMin=[]  SumI1OutMax=[]  SumI2OutMin=[]  SumI2OutMax=[]  SumI3OutMin=[]  SumI3OutMax=[]  SumDOutMin=[]  SumDOutMax=[]  SaturationOutMin=[]  SaturationOutMax=[]  IntegratorContinuousStateAttributes=''  IntegratorStateMustResolveToSignalObject=off  IntegratorRTWStateStorageClass=Auto  FilterContinuousStateAttributes=''  FilterStateMustResolveToSignalObject=off  FilterRTWStateStorageClass=Auto  DifferentiatorICPrevScaledInput=0  DifferentiatorOutMin=[]  DifferentiatorOutMax=[]  FilterDiffOutCoefMin=[]  FilterDiffOutCoefMax=[]  SumDenOutMin=[]  SumDenOutMax=[]  SumNumOutMin=[]  SumNumOutMax=[]  ReciprocalOutMin=[]  ReciprocalOutMax=[]  DivideOutMin=[]  DivideOutMax=[]  TunerSelectOption=Transfer Function Based (PID Tuner App)
  Solenoids : MATLAB Function  TreatAsAtomicUnit=on
  Sum : Sum  Inputs=|+-
  tag scope: L_RF_in=global, L_RF_out=global
  wires:
  Solenoids/3(inside_deadzone_1) -> Delay/1
  Delay/1 -> Solenoids/2(inside_deadzone)
  Pressure Des/1 -> Sum/1
  [L_RF_pres] -> Sum/2
  [L_deadzone_in] -> Solenoids/3(deadzone_in)
  [L_deadzone_out] -> Solenoids/4(deadzone_out)
  Solenoids/1(intake) -> [L_RF_in]
  Solenoids/2(outtake) -> [L_RF_out]
  [L_k_i] -> PID Controller/3
  [L_k_d] -> PID Controller/4
  [L_N] -> PID Controller/5
  Sum/1 -> PID Controller/1
  PID Controller/1 -> Solenoids/1(control)
  [L_k_p] -> PID Controller/2
  [L_PAMs_off] -> Solenoids/5(PAMs_on)
  [System_on] -> Solenoids/6(System_on)
  [L_Depressurize_PAMs] -> Solenoids/7(depressurize)

== system EPA_Walker/PAMs/PAMs Left/SOL ==
  Pressure Des : Inport
  Delay : Delay  DelayLength=1
  PID Controller : simulink/Continuous/PID Controller  Controller=PID  TimeDomain=Discrete-time  SampleTime=-1  IntegratorMethod=Forward Euler  FilterMethod=Forward Euler  Form=Ideal  UseFilter=on  ControllerParametersSource=external  P=k_p_pam  I=0  D=0.45*0.15/8  N=100  InitialConditionSource=internal  InitialConditionForIntegrator=0  InitialConditionForFilter=0  ExternalReset=none  LimitOutput=off  UpperSaturationLimit=inf  LowerSaturationLimit=-inf  LinearizeAsGain=on  AntiWindupMode=none  Kb=1  TrackingMode=off  Kt=1  PParamMin=[]  PParamMax=[]  IParamMin=[]  IParamMax=[]  DParamMin=[]  DParamMax=[]  NParamMin=[]  NParamMax=[]  KbParamMin=[]  KbParamMax=[]  KtParamMin=[]  KtParamMax=[]  POutMin=[]  POutMax=[]  IOutMin=[]  IOutMax=[]  DOutMin=[]  DOutMax=[]  NOutMin=[]  NOutMax=[]  KbOutMin=[]  KbOutMax=[]  KtOutMin=[]  KtOutMax=[]  IntegratorOutMin=[]  IntegratorOutMax=[]  FilterOutMin=[]  FilterOutMax=[]  SumOutMin=[]  SumOutMax=[]  SumI1OutMin=[]  SumI1OutMax=[]  SumI2OutMin=[]  SumI2OutMax=[]  SumI3OutMin=[]  SumI3OutMax=[]  SumDOutMin=[]  SumDOutMax=[]  SaturationOutMin=[]  SaturationOutMax=[]  IntegratorContinuousStateAttributes=''  IntegratorStateMustResolveToSignalObject=off  IntegratorRTWStateStorageClass=Auto  FilterContinuousStateAttributes=''  FilterStateMustResolveToSignalObject=off  FilterRTWStateStorageClass=Auto  DifferentiatorICPrevScaledInput=0  DifferentiatorOutMin=[]  DifferentiatorOutMax=[]  FilterDiffOutCoefMin=[]  FilterDiffOutCoefMax=[]  SumDenOutMin=[]  SumDenOutMax=[]  SumNumOutMin=[]  SumNumOutMax=[]  ReciprocalOutMin=[]  ReciprocalOutMax=[]  DivideOutMin=[]  DivideOutMax=[]  TunerSelectOption=Transfer Function Based (PID Tuner App)
  Solenoids : MATLAB Function  TreatAsAtomicUnit=on
  Sum : Sum  Inputs=|+-
  tag scope: L_SOL_in=global, L_SOL_out=global
  wires:
  Solenoids/3(inside_deadzone_1) -> Delay/1
  Delay/1 -> Solenoids/2(inside_deadzone)
  PID Controller/1 -> Solenoids/1(control)
  Pressure Des/1 -> Sum/1
  [L_SOL_pres] -> Sum/2
  [L_deadzone_in] -> Solenoids/3(deadzone_in)
  [L_deadzone_out] -> Solenoids/4(deadzone_out)
  Solenoids/1(intake) -> [L_SOL_in]
  Solenoids/2(outtake) -> [L_SOL_out]
  [L_k_i] -> PID Controller/3
  [L_k_d] -> PID Controller/4
  [L_N] -> PID Controller/5
  Sum/1 -> PID Controller/1
  [L_k_p] -> PID Controller/2
  [L_PAMs_off] -> Solenoids/5(PAMs_on)
  [System_on] -> Solenoids/6(System_on)
  [L_Depressurize_PAMs] -> Solenoids/7(depressurize)

== system EPA_Walker/PAMs/PAMs Left/TIB ==
  Pressure Des : Inport
  Delay : Delay  DelayLength=1
  PID Controller : simulink/Continuous/PID Controller  Controller=PID  TimeDomain=Discrete-time  SampleTime=-1  IntegratorMethod=Forward Euler  FilterMethod=Forward Euler  Form=Ideal  UseFilter=on  ControllerParametersSource=internal  P=k_p_TIB  I=0  D=0.01  N=300  InitialConditionSource=internal  InitialConditionForIntegrator=0  InitialConditionForFilter=0  ExternalReset=none  LimitOutput=off  UpperSaturationLimit=inf  LowerSaturationLimit=-inf  LinearizeAsGain=on  AntiWindupMode=none  Kb=1  TrackingMode=off  Kt=1  PParamMin=[]  PParamMax=[]  IParamMin=[]  IParamMax=[]  DParamMin=[]  DParamMax=[]  NParamMin=[]  NParamMax=[]  KbParamMin=[]  KbParamMax=[]  KtParamMin=[]  KtParamMax=[]  POutMin=[]  POutMax=[]  IOutMin=[]  IOutMax=[]  DOutMin=[]  DOutMax=[]  NOutMin=[]  NOutMax=[]  KbOutMin=[]  KbOutMax=[]  KtOutMin=[]  KtOutMax=[]  IntegratorOutMin=[]  IntegratorOutMax=[]  FilterOutMin=[]  FilterOutMax=[]  SumOutMin=[]  SumOutMax=[]  SumI1OutMin=[]  SumI1OutMax=[]  SumI2OutMin=[]  SumI2OutMax=[]  SumI3OutMin=[]  SumI3OutMax=[]  SumDOutMin=[]  SumDOutMax=[]  SaturationOutMin=[]  SaturationOutMax=[]  IntegratorContinuousStateAttributes=''  IntegratorStateMustResolveToSignalObject=off  IntegratorRTWStateStorageClass=Auto  FilterContinuousStateAttributes=''  FilterStateMustResolveToSignalObject=off  FilterRTWStateStorageClass=Auto  DifferentiatorICPrevScaledInput=0  DifferentiatorOutMin=[]  DifferentiatorOutMax=[]  FilterDiffOutCoefMin=[]  FilterDiffOutCoefMax=[]  SumDenOutMin=[]  SumDenOutMax=[]  SumNumOutMin=[]  SumNumOutMax=[]  ReciprocalOutMin=[]  ReciprocalOutMax=[]  DivideOutMin=[]  DivideOutMax=[]  TunerSelectOption=Transfer Function Based (PID Tuner App)
  Solenoids : MATLAB Function  TreatAsAtomicUnit=on
  Sum : Sum  Inputs=|+-
  tag scope: L_TIB_in=global, L_TIB_out=global
  wires:
  Solenoids/3(inside_deadzone_1) -> Delay/1
  Delay/1 -> Solenoids/2(inside_deadzone)
  Pressure Des/1 -> Sum/1
  [L_TIB_pres] -> Sum/2
  Solenoids/1(intake) -> [L_TIB_in]
  Solenoids/2(outtake) -> [L_TIB_out]
  [L_PAMs_off] -> Solenoids/3(PAMs_on)
  [System_on] -> Solenoids/4(System_on)
  PID Controller/1 -> Solenoids/1(control)
  Sum/1 -> PID Controller/1
  [L_Depressurize_PAMs] -> Solenoids/5(depressurize)

== system EPA_Walker/PAMs/PAMs Left/VAS ==
  Pressure Des : Inport
  Delay : Delay  DelayLength=1
  PID Controller : simulink/Continuous/PID Controller  Controller=PID  TimeDomain=Discrete-time  SampleTime=-1  IntegratorMethod=Forward Euler  FilterMethod=Forward Euler  Form=Ideal  UseFilter=on  ControllerParametersSource=external  P=k_p_pam  I=0  D=0.45*0.15/8  N=100  InitialConditionSource=internal  InitialConditionForIntegrator=0  InitialConditionForFilter=0  ExternalReset=none  LimitOutput=off  UpperSaturationLimit=inf  LowerSaturationLimit=-inf  LinearizeAsGain=on  AntiWindupMode=none  Kb=1  TrackingMode=off  Kt=1  PParamMin=[]  PParamMax=[]  IParamMin=[]  IParamMax=[]  DParamMin=[]  DParamMax=[]  NParamMin=[]  NParamMax=[]  KbParamMin=[]  KbParamMax=[]  KtParamMin=[]  KtParamMax=[]  POutMin=[]  POutMax=[]  IOutMin=[]  IOutMax=[]  DOutMin=[]  DOutMax=[]  NOutMin=[]  NOutMax=[]  KbOutMin=[]  KbOutMax=[]  KtOutMin=[]  KtOutMax=[]  IntegratorOutMin=[]  IntegratorOutMax=[]  FilterOutMin=[]  FilterOutMax=[]  SumOutMin=[]  SumOutMax=[]  SumI1OutMin=[]  SumI1OutMax=[]  SumI2OutMin=[]  SumI2OutMax=[]  SumI3OutMin=[]  SumI3OutMax=[]  SumDOutMin=[]  SumDOutMax=[]  SaturationOutMin=[]  SaturationOutMax=[]  IntegratorContinuousStateAttributes=''  IntegratorStateMustResolveToSignalObject=off  IntegratorRTWStateStorageClass=Auto  FilterContinuousStateAttributes=''  FilterStateMustResolveToSignalObject=off  FilterRTWStateStorageClass=Auto  DifferentiatorICPrevScaledInput=0  DifferentiatorOutMin=[]  DifferentiatorOutMax=[]  FilterDiffOutCoefMin=[]  FilterDiffOutCoefMax=[]  SumDenOutMin=[]  SumDenOutMax=[]  SumNumOutMin=[]  SumNumOutMax=[]  ReciprocalOutMin=[]  ReciprocalOutMax=[]  DivideOutMin=[]  DivideOutMax=[]  TunerSelectOption=Transfer Function Based (PID Tuner App)
  Solenoids : MATLAB Function  TreatAsAtomicUnit=on
  Sum : Sum  Inputs=|+-
  tag scope: L_VAS_in=global, L_VAS_out=global
  wires:
  Solenoids/3(inside_deadzone_1) -> Delay/1
  Delay/1 -> Solenoids/2(inside_deadzone)
  Pressure Des/1 -> Sum/1
  [L_VAS_pres] -> Sum/2
  [L_deadzone_in] -> Solenoids/3(deadzone_in)
  [L_deadzone_out] -> Solenoids/4(deadzone_out)
  Solenoids/1(intake) -> [L_VAS_in]
  [L_k_i] -> PID Controller/3
  [L_k_d] -> PID Controller/4
  [L_N] -> PID Controller/5
  Sum/1 -> PID Controller/1
  PID Controller/1 -> Solenoids/1(control)
  [L_k_p] -> PID Controller/2
  [L_PAMs_off] -> Solenoids/5(PAMs_on)
  [System_on] -> Solenoids/6(System_on)
  Solenoids/2(outtake) -> [L_VAS_out]
  [L_Depressurize_PAMs] -> Solenoids/7(depressurize)

== system EPA_Walker/PAMs/PAMs Right/GAS ==
  Pressure Des : Inport
  Delay : Delay  DelayLength=1
  PID Controller : simulink/Continuous/PID Controller  Controller=PID  TimeDomain=Discrete-time  SampleTime=-1  IntegratorMethod=Forward Euler  FilterMethod=Forward Euler  Form=Ideal  UseFilter=on  ControllerParametersSource=external  P=k_p_pam  I=0  D=0.45*0.15/8  N=100  InitialConditionSource=internal  InitialConditionForIntegrator=0  InitialConditionForFilter=0  ExternalReset=none  LimitOutput=off  UpperSaturationLimit=inf  LowerSaturationLimit=-inf  LinearizeAsGain=on  AntiWindupMode=none  Kb=1  TrackingMode=off  Kt=1  PParamMin=[]  PParamMax=[]  IParamMin=[]  IParamMax=[]  DParamMin=[]  DParamMax=[]  NParamMin=[]  NParamMax=[]  KbParamMin=[]  KbParamMax=[]  KtParamMin=[]  KtParamMax=[]  POutMin=[]  POutMax=[]  IOutMin=[]  IOutMax=[]  DOutMin=[]  DOutMax=[]  NOutMin=[]  NOutMax=[]  KbOutMin=[]  KbOutMax=[]  KtOutMin=[]  KtOutMax=[]  IntegratorOutMin=[]  IntegratorOutMax=[]  FilterOutMin=[]  FilterOutMax=[]  SumOutMin=[]  SumOutMax=[]  SumI1OutMin=[]  SumI1OutMax=[]  SumI2OutMin=[]  SumI2OutMax=[]  SumI3OutMin=[]  SumI3OutMax=[]  SumDOutMin=[]  SumDOutMax=[]  SaturationOutMin=[]  SaturationOutMax=[]  IntegratorContinuousStateAttributes=''  IntegratorStateMustResolveToSignalObject=off  IntegratorRTWStateStorageClass=Auto  FilterContinuousStateAttributes=''  FilterStateMustResolveToSignalObject=off  FilterRTWStateStorageClass=Auto  DifferentiatorICPrevScaledInput=0  DifferentiatorOutMin=[]  DifferentiatorOutMax=[]  FilterDiffOutCoefMin=[]  FilterDiffOutCoefMax=[]  SumDenOutMin=[]  SumDenOutMax=[]  SumNumOutMin=[]  SumNumOutMax=[]  ReciprocalOutMin=[]  ReciprocalOutMax=[]  DivideOutMin=[]  DivideOutMax=[]  TunerSelectOption=Transfer Function Based (PID Tuner App)
  Solenoids : MATLAB Function  TreatAsAtomicUnit=on
  Sum : Sum  Inputs=|+-
  tag scope: R_GAS_in=global, R_GAS_out=global
  wires:
  Solenoids/3(inside_deadzone_1) -> Delay/1
  Delay/1 -> Solenoids/2(inside_deadzone)
  Pressure Des/1 -> Sum/1
  [R_GAS_pres] -> Sum/2
  [R_deadzone_in] -> Solenoids/3(deadzone_in)
  [R_deadzone_out] -> Solenoids/4(deadzone_out)
  Solenoids/1(intake) -> [R_GAS_in]
  Solenoids/2(outtake) -> [R_GAS_out]
  [R_k_i] -> PID Controller/3
  [R_k_d] -> PID Controller/4
  [R_N] -> PID Controller/5
  Sum/1 -> PID Controller/1
  PID Controller/1 -> Solenoids/1(control)
  [R_k_p] -> PID Controller/2
  [R_PAMs_off] -> Solenoids/5(PAMs_on)
  [System_on] -> Solenoids/6(System_on)
  [R_Depressurize_PAMs] -> Solenoids/7(depressurize)

== system EPA_Walker/PAMs/PAMs Right/GL ==
  Pressure Des : Inport
  Delay : Delay  DelayLength=1
  PID Controller : simulink/Continuous/PID Controller  Controller=PID  TimeDomain=Discrete-time  SampleTime=-1  IntegratorMethod=Forward Euler  FilterMethod=Forward Euler  Form=Ideal  UseFilter=on  ControllerParametersSource=external  P=k_p_pam  I=0  D=0.45*0.15/8  N=100  InitialConditionSource=internal  InitialConditionForIntegrator=0  InitialConditionForFilter=0  ExternalReset=none  LimitOutput=off  UpperSaturationLimit=inf  LowerSaturationLimit=-inf  LinearizeAsGain=on  AntiWindupMode=none  Kb=1  TrackingMode=off  Kt=1  PParamMin=[]  PParamMax=[]  IParamMin=[]  IParamMax=[]  DParamMin=[]  DParamMax=[]  NParamMin=[]  NParamMax=[]  KbParamMin=[]  KbParamMax=[]  KtParamMin=[]  KtParamMax=[]  POutMin=[]  POutMax=[]  IOutMin=[]  IOutMax=[]  DOutMin=[]  DOutMax=[]  NOutMin=[]  NOutMax=[]  KbOutMin=[]  KbOutMax=[]  KtOutMin=[]  KtOutMax=[]  IntegratorOutMin=[]  IntegratorOutMax=[]  FilterOutMin=[]  FilterOutMax=[]  SumOutMin=[]  SumOutMax=[]  SumI1OutMin=[]  SumI1OutMax=[]  SumI2OutMin=[]  SumI2OutMax=[]  SumI3OutMin=[]  SumI3OutMax=[]  SumDOutMin=[]  SumDOutMax=[]  SaturationOutMin=[]  SaturationOutMax=[]  IntegratorContinuousStateAttributes=''  IntegratorStateMustResolveToSignalObject=off  IntegratorRTWStateStorageClass=Auto  FilterContinuousStateAttributes=''  FilterStateMustResolveToSignalObject=off  FilterRTWStateStorageClass=Auto  DifferentiatorICPrevScaledInput=0  DifferentiatorOutMin=[]  DifferentiatorOutMax=[]  FilterDiffOutCoefMin=[]  FilterDiffOutCoefMax=[]  SumDenOutMin=[]  SumDenOutMax=[]  SumNumOutMin=[]  SumNumOutMax=[]  ReciprocalOutMin=[]  ReciprocalOutMax=[]  DivideOutMin=[]  DivideOutMax=[]  TunerSelectOption=Transfer Function Based (PID Tuner App)
  Solenoids : MATLAB Function  TreatAsAtomicUnit=on
  Sum : Sum  Inputs=|+-
  tag scope: R_GL_in=global, R_GL_out=global
  wires:
  Solenoids/3(inside_deadzone_1) -> Delay/1
  Delay/1 -> Solenoids/2(inside_deadzone)
  Pressure Des/1 -> Sum/1
  [R_GL_pres] -> Sum/2
  [R_deadzone_in] -> Solenoids/3(deadzone_in)
  [R_deadzone_out] -> Solenoids/4(deadzone_out)
  Solenoids/1(intake) -> [R_GL_in]
  Solenoids/2(outtake) -> [R_GL_out]
  [R_k_i] -> PID Controller/3
  [R_k_d] -> PID Controller/4
  [R_N] -> PID Controller/5
  Sum/1 -> PID Controller/1
  PID Controller/1 -> Solenoids/1(control)
  [R_k_p] -> PID Controller/2
  [R_PAMs_off] -> Solenoids/5(PAMs_on)
  [System_on] -> Solenoids/6(System_on)
  [R_Depressurize_PAMs] -> Solenoids/7(depressurize)

== system EPA_Walker/PAMs/PAMs Right/HAM ==
  Pressure Des : Inport
  Delay : Delay  DelayLength=1
  PID Controller : simulink/Continuous/PID Controller  Controller=PID  TimeDomain=Discrete-time  SampleTime=-1  IntegratorMethod=Forward Euler  FilterMethod=Forward Euler  Form=Ideal  UseFilter=on  ControllerParametersSource=external  P=k_p_pam  I=0  D=0.45*0.15/8  N=100  InitialConditionSource=internal  InitialConditionForIntegrator=0  InitialConditionForFilter=0  ExternalReset=none  LimitOutput=off  UpperSaturationLimit=inf  LowerSaturationLimit=-inf  LinearizeAsGain=on  AntiWindupMode=none  Kb=1  TrackingMode=off  Kt=1  PParamMin=[]  PParamMax=[]  IParamMin=[]  IParamMax=[]  DParamMin=[]  DParamMax=[]  NParamMin=[]  NParamMax=[]  KbParamMin=[]  KbParamMax=[]  KtParamMin=[]  KtParamMax=[]  POutMin=[]  POutMax=[]  IOutMin=[]  IOutMax=[]  DOutMin=[]  DOutMax=[]  NOutMin=[]  NOutMax=[]  KbOutMin=[]  KbOutMax=[]  KtOutMin=[]  KtOutMax=[]  IntegratorOutMin=[]  IntegratorOutMax=[]  FilterOutMin=[]  FilterOutMax=[]  SumOutMin=[]  SumOutMax=[]  SumI1OutMin=[]  SumI1OutMax=[]  SumI2OutMin=[]  SumI2OutMax=[]  SumI3OutMin=[]  SumI3OutMax=[]  SumDOutMin=[]  SumDOutMax=[]  SaturationOutMin=[]  SaturationOutMax=[]  IntegratorContinuousStateAttributes=''  IntegratorStateMustResolveToSignalObject=off  IntegratorRTWStateStorageClass=Auto  FilterContinuousStateAttributes=''  FilterStateMustResolveToSignalObject=off  FilterRTWStateStorageClass=Auto  DifferentiatorICPrevScaledInput=0  DifferentiatorOutMin=[]  DifferentiatorOutMax=[]  FilterDiffOutCoefMin=[]  FilterDiffOutCoefMax=[]  SumDenOutMin=[]  SumDenOutMax=[]  SumNumOutMin=[]  SumNumOutMax=[]  ReciprocalOutMin=[]  ReciprocalOutMax=[]  DivideOutMin=[]  DivideOutMax=[]  TunerSelectOption=Transfer Function Based (PID Tuner App)
  Solenoids : MATLAB Function  TreatAsAtomicUnit=on
  Sum : Sum  Inputs=|+-
  tag scope: R_HAM_in=global, R_HAM_out=global
  wires:
  Solenoids/3(inside_deadzone_1) -> Delay/1
  Delay/1 -> Solenoids/2(inside_deadzone)
  Pressure Des/1 -> Sum/1
  [R_HAM_pres] -> Sum/2
  [R_deadzone_in] -> Solenoids/3(deadzone_in)
  [R_deadzone_out] -> Solenoids/4(deadzone_out)
  Solenoids/1(intake) -> [R_HAM_in]
  Solenoids/2(outtake) -> [R_HAM_out]
  [R_k_i] -> PID Controller/3
  [R_k_d] -> PID Controller/4
  [R_N] -> PID Controller/5
  Sum/1 -> PID Controller/1
  PID Controller/1 -> Solenoids/1(control)
  [R_k_p] -> PID Controller/2
  [R_PAMs_off] -> Solenoids/5(PAMs_on)
  [System_on] -> Solenoids/6(System_on)
  [R_Depressurize_PAMs] -> Solenoids/7(depressurize)
